simulink model "ballbeam_sim1"  (R2016b)
settings: Solver=ode45  StartTime=0.0  StopTime=P.t_end  RelTol=1e-3  EnableMultiTasking=on
InitFcn:
  | addpath ./..
  | ballbeam_param
  | ballbeamParamHW10
undefined symbols (not defined in the file or in its folder): ballbeam_animation, ballbeam_ctrl, P
settings Model: Creator=beard  LastModifiedBy=beard
settings DataIOCC: LimitDataPoints=on  SaveFormat=Array  SignalLoggingSaveFormat=ModelDataLogs
settings OptimizationCC: ExpressionDepthLimit=2147483647  InitFltsAndDblsToZero=on  LifeSpan=inf
settings DebuggingCC: UnderspecifiedInitializationDetection=Classic  MergeDetectMultiDrivingBlocksExec=none  SolverPrmCheckMsg=warning  FcnCallInpInsideContextMsg=warning  StateNameClashWarn=warning  SFUnexpectedBacktrackingDiag=warning  SFNoUnconditionalDefaultTransitionDiag=warning  SFExecutionAtInitializationDiag=none
settings HardwareCC: ProdBitPerPointer=32  ProdBitPerSizeT=32  ProdBitPerPtrDiffT=32  ProdLargestAtomicFloat=None  ProdIntDivRoundTo=Undefined  ProdEndianess=Unspecified  ProdWordSize=32  ProdHWDeviceType=32-bit Generic
settings ModelReferenceCC: PropagateSignalLabelsOutOfModel=off
settings GRTTargetCC: TargetLangStandard=C89/C90 (ANSI)  GeneratePreprocessorConditionals=Disable all  CombineOutputUpdateFcns=off  GRTInterface=on
settings ConfigComp: CovMetricSettings=dw  CovHtmlReporting=on  CovSaveCumulativeToWorkspaceVar=on  CovSaveSingleToWorkspaceVar=on  CovExternalEMLEnable=off

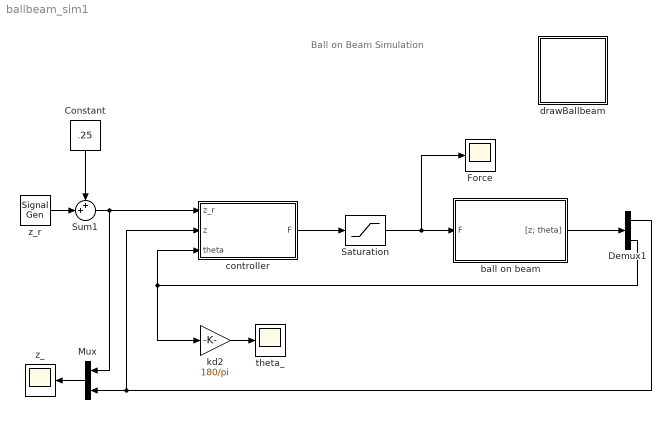
== system ballbeam_sim1 ==
  note: Ball on Beam Simulation
  Constant : Constant  Value=.25
  Demux1 : Demux  Outputs=2
  Force : Scope
  Mux : Mux  Inputs=2
  Saturation : Saturate  UpperLimit=P.Fmax  LowerLimit=-P.Fmax
  Sum1 : Sum  Inputs=++|
  ball on beam : Subsystem
  controller : Subsystem
  drawBallbeam : Subsystem
      mask Display: image(imread('tv.jpg'))
  kd2 : Gain  Gain=180/pi
  theta_ : Scope
  z_ : Scope
  z_r : SignalGenerator  WaveForm=square  Amplitude=0.125  Frequency=.04
  wires:
  z_r/1 -> Sum1/2
  Constant/1 -> Sum1/1
  controller/1(F) -> Saturation/1
  ball on beam/1("[z; theta]") -> Demux1/1
  Demux1/2 -> controller/3(theta), kd2/1
  Demux1/1 -> controller/2(z), Mux/2
  Mux/1 -> z_/1
  kd2/1 -> theta_/1
  Sum1/1 -> controller/1(z_r), Mux/1
  Saturation/1 -> ball on beam/1(F), Force/1

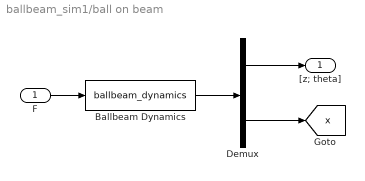
== system ballbeam_sim1/ball on beam ==
  F : Inport
  Ballbeam Dynamics : S-Function  FunctionName=ballbeam_dynamics  Parameters=P  SFunctionDeploymentMode=off  EnableBusSupport=off
  Demux : Demux  Outputs=[2;4]
  "[z; theta]" : Outport
  tag scope: x=global
  wires:
  Demux/2 -> [x]
  Demux/1 -> "[z; theta]"/1
  Ballbeam Dynamics/1 -> Demux/1
  F/1 -> Ballbeam Dynamics/1

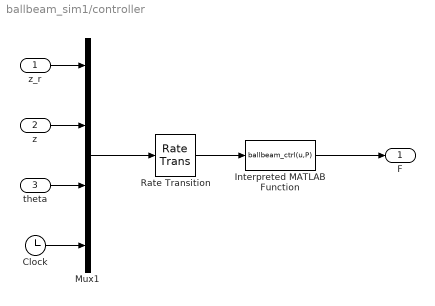
== system ballbeam_sim1/controller ==
  z_r : Inport
  z : Inport  Port=2
  theta : Inport  Port=3
  Clock : Clock
  Interpreted MATLAB Function : MATLABFcn  MATLABFcn=ballbeam_ctrl(u,P)  OutputDimensions=1
  Mux1 : Mux
  Rate Transition : RateTransition  OutPortSampleTime=P.Ts
  F : Outport
  wires:
  Mux1/1 -> Rate Transition/1
  z_r/1 -> Mux1/1
  Interpreted MATLAB Function/1 -> F/1
  Clock/1 -> Mux1/4
  Rate Transition/1 -> Interpreted MATLAB Function/1
  theta/1 -> Mux1/3
  z/1 -> Mux1/2

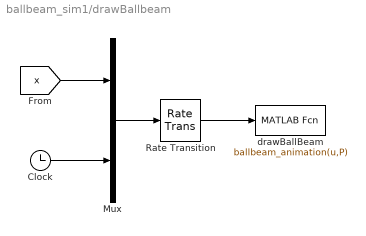
== system ballbeam_sim1/drawBallbeam ==
  Clock : Clock
  Mux : Mux  Inputs=2
  Rate Transition : RateTransition  OutPortSampleTime=P.t_plot
  drawBallBeam : MATLABFcn  MATLABFcn=ballbeam_animation(u,P)  OutputDimensions=0
  wires:
  Mux/1 -> Rate Transition/1
  [x] -> Mux/1
  Clock/1 -> Mux/2
  Rate Transition/1 -> drawBallBeam/1
